simulink model "Traslational_Motion_Observer_2"  (R2016b)
settings: Solver=VariableStepAuto  StartTime=0.0  StopTime=10.0  RelTol=1e-3
settings Model: Creator=liana  LastModifiedBy=liana

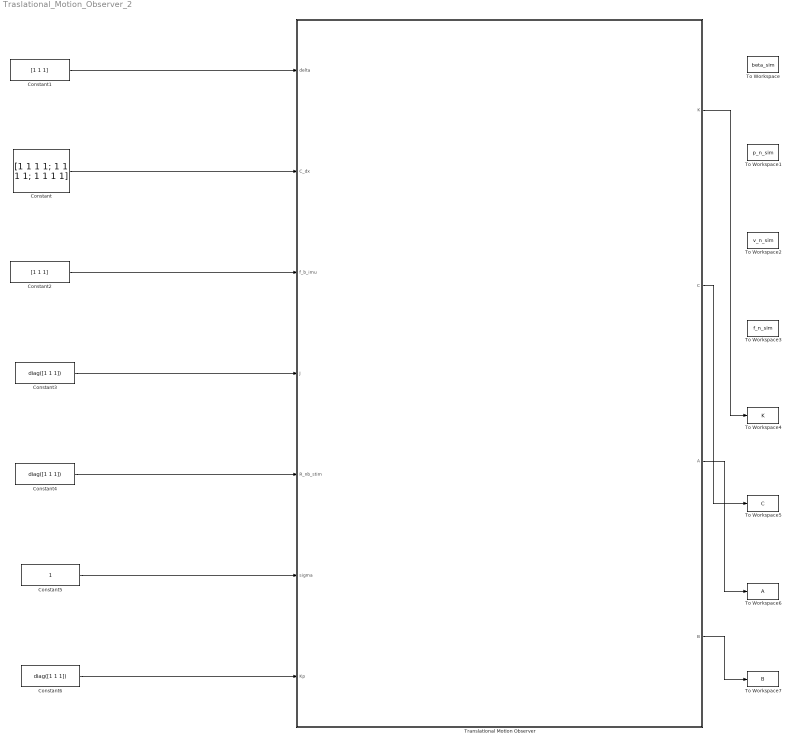
== system Traslational_Motion_Observer_2 ==
  Constant : Constant  Value=[1 1 1 1; 1 1 1 1; 1 1 1 1]
  Constant1 : Constant  Value=[1 1 1]
  Constant2 : Constant  Value=[1 1 1]
  Constant3 : Constant  Value=diag([1 1 1])
  Constant4 : Constant  Value=diag([1 1 1])
  Constant5 : Constant
  Constant6 : Constant  Value=diag([1 1 1])
  To Workspace : ToWorkspace  VariableName=beta_sim  SampleTime=-1
  To Workspace1 : ToWorkspace  VariableName=p_n_sim  SampleTime=-1
  To Workspace2 : ToWorkspace  VariableName=v_n_sim  SampleTime=-1
  To Workspace3 : ToWorkspace  VariableName=f_n_sim  SampleTime=-1
  To Workspace4 : ToWorkspace  VariableName=K  SampleTime=-1
  To Workspace5 : ToWorkspace  VariableName=C  SampleTime=-1
  To Workspace6 : ToWorkspace  VariableName=A  SampleTime=-1
  To Workspace7 : ToWorkspace  VariableName=B  SampleTime=-1
  Translational Motion Observer : Subsystem
  wires:
  ? -> To Workspace/1
  ? -> To Workspace1/1
  ? -> To Workspace2/1
  ? -> To Workspace3/1
  Translational Motion Observer/1(K) -> To Workspace4/1
  Translational Motion Observer/2("C ") -> To Workspace5/1
  Translational Motion Observer/3(" A") -> To Workspace6/1
  Translational Motion Observer/4(B) -> To Workspace7/1
  Constant/1 -> Translational Motion Observer/2(C_dx)
  Constant1/1 -> Translational Motion Observer/1(delta)
  Constant2/1 -> Translational Motion Observer/3(f_b_imu)
  Constant3/1 -> Translational Motion Observer/4(J)
  Constant4/1 -> Translational Motion Observer/5(R_nb_stim)
  Constant5/1 -> Translational Motion Observer/6(sigma)
  Constant6/1 -> Translational Motion Observer/7(Kp)

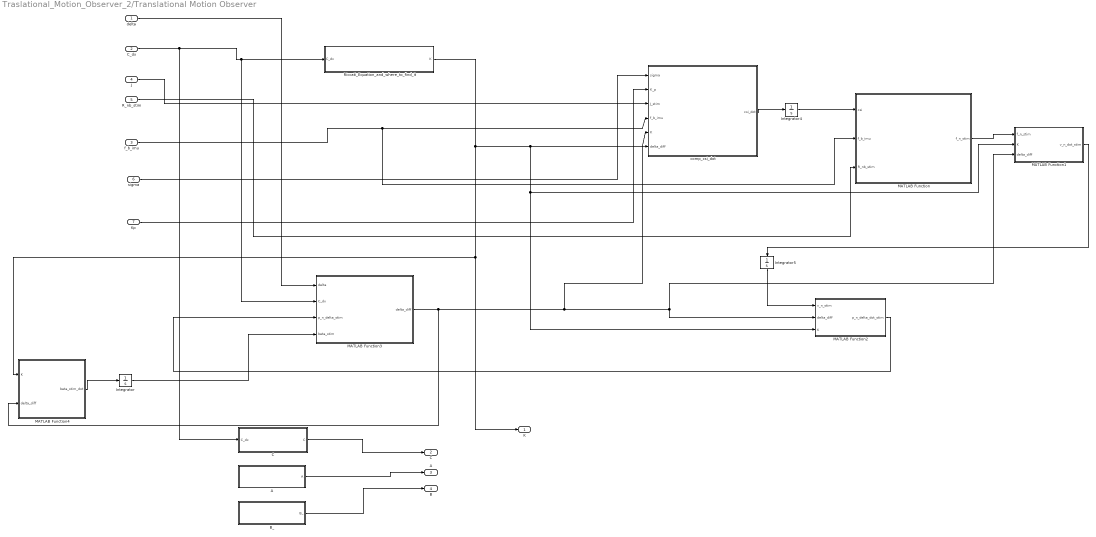
== system Traslational_Motion_Observer_2/Translational Motion Observer ==
  delta : Inport
  C_dx : Inport  Port=2
  f_b_imu : Inport  Port=3
  J : Inport  Port=4
  R_nb_stim : Inport  Port=5
  sigma : Inport  Port=6
  Kp : Inport  Port=7
  A : MATLAB Function  TreatAsAtomicUnit=on
  B_ : MATLAB Function  TreatAsAtomicUnit=on
  C : MATLAB Function  TreatAsAtomicUnit=on
  Integrator : Integrator
  Integrator4 : Integrator
  Integrator5 : Integrator
  MATLAB Function : MATLAB Function  TreatAsAtomicUnit=on
  MATLAB Function1 : MATLAB Function  TreatAsAtomicUnit=on
  MATLAB Function2 : MATLAB Function  TreatAsAtomicUnit=on
  MATLAB Function3 : MATLAB Function  TreatAsAtomicUnit=on
  MATLAB Function4 : MATLAB Function  TreatAsAtomicUnit=on
  Riccati_Equation_and_where_to_find_it : Subsystem
  comp_csi_dot : MATLAB Function  TreatAsAtomicUnit=on
  K : Outport
  "C " : Outport  Port=2
  " A" : Outport  Port=3
  B : Outport  Port=4
  wires:
  C_dx/1 -> C/1(C_dx), MATLAB Function3/2(C_dx), Riccati_Equation_and_where_to_find_it/1(C_dx)
  sigma/1 -> comp_csi_dot/1(sigma)
  A/1(A) -> " A"/1
  C/1(C) -> "C "/1
  Riccati_Equation_and_where_to_find_it/1(K) -> MATLAB Function2/3(K), MATLAB Function1/2(K), comp_csi_dot/5(K), MATLAB Function4/1(K), K/1
  B_/1(B_) -> B/1
  comp_csi_dot/1(csi_dot) -> Integrator4/1
  Integrator4/1 -> MATLAB Function/1(csi)
  MATLAB Function/1(f_n_stim) -> MATLAB Function1/1(f_n_stim)
  MATLAB Function1/1(v_n_dot_stim) -> Integrator5/1
  Integrator5/1 -> MATLAB Function2/1(v_n_stim)
  Kp/1 -> comp_csi_dot/2(K_p)
  J/1 -> comp_csi_dot/3(J_stim)
  f_b_imu/1 -> MATLAB Function/2(f_b_imu), comp_csi_dot/4(f_b_imu)
  R_nb_stim/1 -> MATLAB Function/3(R_nb_stim)
  MATLAB Function3/1(delta_diff) -> MATLAB Function4/2(delta_diff), comp_csi_dot/6(delta_diff), MATLAB Function1/3(delta_diff), MATLAB Function2/2(delta_diff)
  MATLAB Function2/1(p_n_delta_dot_stim) -> MATLAB Function3/3(p_n_delta_stim)
  delta/1 -> MATLAB Function3/1(delta)
  MATLAB Function4/1(beta_stim_dot) -> Integrator/1
  Integrator/1 -> MATLAB Function3/4(beta_stim)

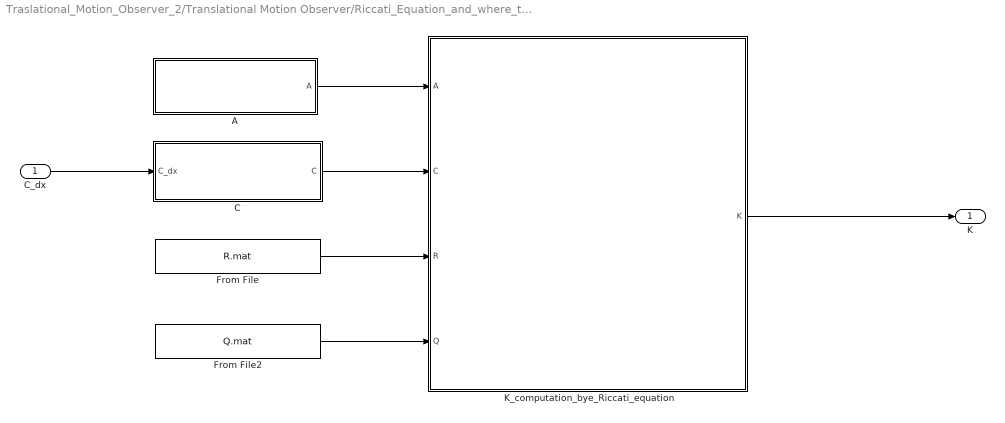
== system Traslational_Motion_Observer_2/Translational Motion Observer/Riccati_Equation_and_where_to_find_it ==
  C_dx : Inport
  A : MATLAB Function  TreatAsAtomicUnit=on
  C : MATLAB Function  TreatAsAtomicUnit=on
  From File : FromFile  FileName=R.mat  SampleTime=0
  From File2 : FromFile  FileName=Q.mat  SampleTime=0
  K_computation_bye_Riccati_equation : MATLAB Function  TreatAsAtomicUnit=on
  K : Outport
  wires:
  C_dx/1 -> C/1(C_dx)
  K_computation_bye_Riccati_equation/1(K) -> K/1
  From File/1 -> K_computation_bye_Riccati_equation/3(R)
  A/1(A) -> K_computation_bye_Riccati_equation/1(A)
  From File2/1 -> K_computation_bye_Riccati_equation/4(Q)
  C/1(C) -> K_computation_bye_Riccati_equation/2(C)

== matlab function Traslational_Motion_Observer_2/Translational Motion Observer/MATLAB Function1 ==
  data: f_n_stim input; v_n_dot_stim output; K input; delta_diff input
function v_n_dot_stim = compute_v_n_dot_stim(f_n_stim, K, delta_diff)

    %Eq. 16
    
    K_v_p = K(5:7,:);
    g_n = [0 0 9.81]';
    v_n_dot_stim  = f_n_stim + g_n + K_v_p*delta_diff;

end

== matlab function Traslational_Motion_Observer_2/Translational Motion Observer/comp_csi_dot ==
  data: sigma input; csi_dot output; K_p input; J_stim input; f_b_imu input; K input; delta_diff input
function csi_dot = compute_csi_dot(sigma,K_p, J_stim, f_b_imu, K, delta_diff)

    %Eq. 17
    
    K_csi_p = K(8:10,:);

    csi_dot   = -sigma*K_p*J_stim*f_b_imu + K_csi_p*delta_diff;

end

== matlab function Traslational_Motion_Observer_2/Translational Motion Observer/MATLAB Function ==
  data: csi input; f_n_stim output; f_b_imu input; R_nb_stim input
function f_n_stim = cpmpute_f_n_stim(csi, f_b_imu, R_nb_stim)

    %Eq. 18

    f_n_stim = R_nb_stim*f_b_imu + csi;

end

== matlab function Traslational_Motion_Observer_2/Translational Motion Observer/MATLAB Function2 ==
  data: v_n_stim input; p_n_delta_dot_stim output; delta_diff input; K input
function p_n_delta_dot_stim = compute_p_n_delta_dot_stim(v_n_stim, delta_diff, K)

    K_pp = K(1:3,:);
    p_n_delta_dot_stim = v_n_stim + K_pp * delta_diff;        % eq 14

end

== matlab function Traslational_Motion_Observer_2/Translational Motion Observer/MATLAB Function3 ==
  data: delta input; delta_diff output; C_dx input; p_n_delta_stim input; beta_stim input
function delta_diff = compute_delta_diff(delta, C_dx, p_n_delta_stim, beta_stim)

    x_stim = [p_n_delta_stim; beta_stim];
    
    delta_stim = 2*C_dx*x_stim;
    
    delta_diff = delta - delta_stim;

end

== matlab function Traslational_Motion_Observer_2/Translational Motion Observer/MATLAB Function4 ==
  data: K input; beta_stim_dot output; delta_diff input
function beta_stim_dot = compute_beta_stim_dot(K, delta_diff)

    %eq. 15
     K_beta_p = K(4,:);
     beta_stim_dot = K_beta_p * delta_diff;

end

== matlab function Traslational_Motion_Observer_2/Translational Motion Observer/Riccati_Equation_and_where_to_find_it/K_computation_bye_Riccati_equation ==
  data: A input; K output; C input; R input; Q input
function K = K_func(A,C,R,Q)

K = zeros(10,3);

coder.extrinsic('care');

[P,L,G] = care(A,C',Q,R);

R_inv = pinv(R); 

K = P*C'*R_inv;

== matlab function Traslational_Motion_Observer_2/Translational Motion Observer/Riccati_Equation_and_where_to_find_it/A ==
  data: A output
function A = A()

 A = zeros(10);

 A(1:3,5:7) = eye(3);
 A(5:7,8:10) = eye(3);
 
A;

== matlab function Traslational_Motion_Observer_2/Translational Motion Observer/Riccati_Equation_and_where_to_find_it/C ==
  data: C output; C_dx input
function C = C(C_dx)

   row = size(C_dx,1); 

   C1 = zeros(row,6);

 C = [2*C_dx C1];

== matlab function Traslational_Motion_Observer_2/Translational Motion Observer/A ==
  data: A output
function A = A()

 A = zeros(10);

 A(1:3,5:7) = eye(3);
 A(5:7,8:10) = eye(3);
 
end

== matlab function Traslational_Motion_Observer_2/Translational Motion Observer/C ==
  data: C output; C_dx input
function C = C(C_dx)

   row = size(C_dx,1); 

   C1 = zeros(row,6);

 C = [2*C_dx C1];
 
 
end

== matlab function Traslational_Motion_Observer_2/Translational Motion Observer/B_ ==
  data: B_ output
function B_ = B()

 B_ = zeros(10,3);

 B_(8:10,1:3) = eye(3);
end
